simulink model "SIR_sim"  (R2023b)
settings: Solver=VariableStepAuto  StartTime=0.0  StopTime=1000  RelTol=1e-3
settings Model: Creator=stefa  LastModifiedBy=stefa

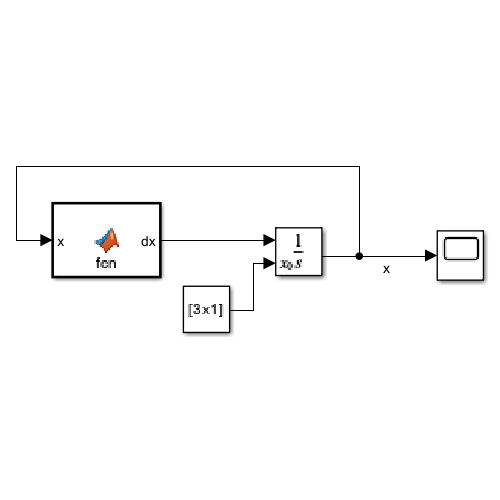
[thumbnail: Simulink's stored preview of the top-level diagram]
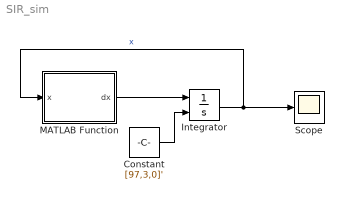
== system SIR_sim ==
  Constant : Constant  Value=[97,3,0]'
  Integrator : Integrator  InitialConditionSource=external
  MATLAB Function : MATLAB Function  TreatAsAtomicUnit=on
  Scope : Scope
  wires:
  MATLAB Function/1(dx) -> Integrator/1
  Constant/1 -> Integrator/2
  Integrator/1 -> Scope/1, MATLAB Function/1(x)  "x"

== matlab function SIR_sim/MATLAB Function ==
  data: dx output; x input
function dx = fcn(x)


b=0.004;     %probabilità di incontro e capacità contagio
g=0.04;      % velocità con cui gli ifetti guariscono
u=1e-3;      % tasso di mortalità altre cause
d=0.01;      % tasso di mortalità causa virus

S=x(1);
I=x(2);
R=x(3);

dx=[ -b*S*I-u*S;
    b*S*I-g*I-u*I;
    g*I-u*R];
